simulink model "F16nonlin_K_q"  (R2023b)
settings: Solver=ode4  StartTime=0  StopTime=5  FixedStep=0.01  RelTol=1e-3  EnableMultiTasking=on
values from neighbouring files (symbols this model uses):
  C_nl = C(8,:)    [compare_lin_nonlin.m]    (also in plot_Kq_lin_nonlin.m; runsim_K_pqr.m)
  CA_nl = C_nl*A    [compare_lin_nonlin.m]    (also in plot_Kq_lin_nonlin.m; runsim_K_pqr.m)
  fc = 1/2    (= 0.5)    [compare_lin_nonlin.m]    (also in plot_Kq_lin_nonlin.m)
  invCB_nl = inv(CB_nl)    [compare_lin_nonlin.m]    (also in plot_Kq_lin_nonlin.m; runsim_K_pqr.m)
  Kq = 2    [compare_lin_nonlin.m]    (also in plot_Kq_lin_nonlin.m)
  U_trim = [0.154007747083 -0.694801754663 0.00182544197392 0.000329744079809]    [trimcond.mat]
  X_trim = [501.999976668 0.0505473192089 -2.30406790676e-05 0.000102787556036 0.0505344970072 7.11881239542e-07 -0.000134428882921 -3.64533551716e-06 -1.91663482729e-05 0 0 0 ... (13 elements, 13x1)]    [trimcond.mat]
  xcg = 0.35    [trimcond.mat]
settings Model: Creator=keviczky  LastModifiedBy=suvo
settings DataIOCC: Decimation=50  SaveFormat=Array  SignalLoggingSaveFormat=ModelDataLogs  ReturnWorkspaceOutputs=off  SignalLoggingName=sigsOut
settings OptimizationCC: BooleanDataType=off
settings DebuggingCC: SaveWithParameterizedLinksMsg=none  UnderspecifiedInitializationDetection=Classic  MergeDetectMultiDrivingBlocksExec=none  SignalResolutionControl=TryResolveAllWithWarning  MultiTaskDSMMsg=warning  MultiTaskCondExecSysMsg=none  UnconnectedInputMsg=warning  UnconnectedOutputMsg=warning  UnconnectedLineMsg=warning
settings HardwareCC: ProdBitPerPointer=32  ProdBitPerSizeT=32  ProdBitPerPtrDiffT=32  ProdLargestAtomicFloat=None  ProdIntDivRoundTo=Undefined  ProdEndianess=Unspecified  ProdWordSize=32  ProdHWDeviceType=32-bit Generic  TargetUnknown=on
settings ModelReferenceCC: PropagateSignalLabelsOutOfModel=off
settings GRTTargetCC: CombineOutputUpdateFcns=off  GRTInterface=on
settings ConfigComp: CovMetricSettings=dw  CovSaveCumulativeToWorkspaceVar=on  CovSaveSingleToWorkspaceVar=on

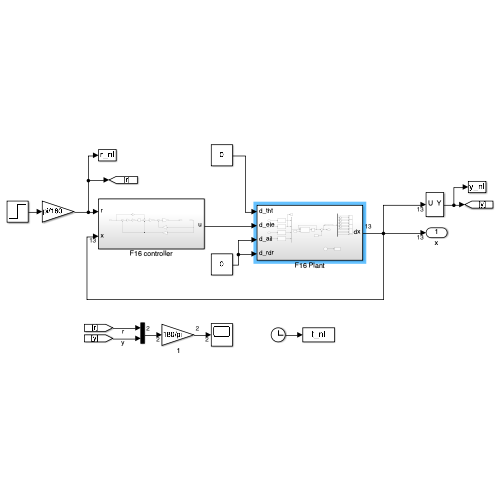
[thumbnail: Simulink's stored preview of the top-level diagram]
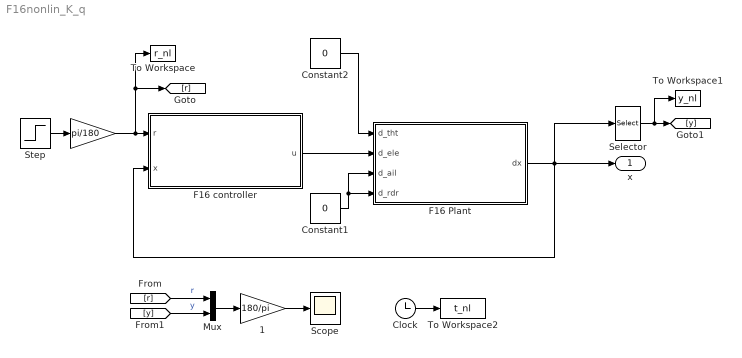
== system F16nonlin_K_q ==
  " " : Gain  Gain=pi/180
  " 1" : Gain  Gain=180/pi
  Clock : Clock
  Constant1 : Constant  Value=0
  Constant2 : Constant  Value=0
  F16 Plant : Subsystem
  F16 controller : Subsystem
  Mux : Mux  Inputs=2
  Scope : Scope
  Selector : Selector  InputPortWidth=13  IndexOptions=Index vector (dialog)  Indices=8  OutputSizes=1
  Step : Step  SampleTime=0
  To Workspace : ToWorkspace  VariableName=r_nl  SampleTime=-1
  To Workspace1 : ToWorkspace  VariableName=y_nl  SampleTime=-1
  To Workspace2 : ToWorkspace  VariableName=t_nl  SampleTime=-1
  x : Outport
  wires:
  Constant2/1 -> F16 Plant/1(d_tht)
  Step/1 -> " "/1
  [r] -> Mux/1  "r"
  [y] -> Mux/2  "y"
  Mux/1 -> " 1"/1
  Selector/1 -> To Workspace1/1, [y]
  " "/1 -> F16 controller/1(r), To Workspace/1, [r]
  " 1"/1 -> Scope/1
  Clock/1 -> To Workspace2/1
  Constant1/1 -> F16 Plant/4(d_rdr), F16 Plant/3(d_ail)
  F16 Plant/1(dx) -> F16 controller/2(x), Selector/1, x/1
  F16 controller/1(u) -> F16 Plant/2(d_ele)

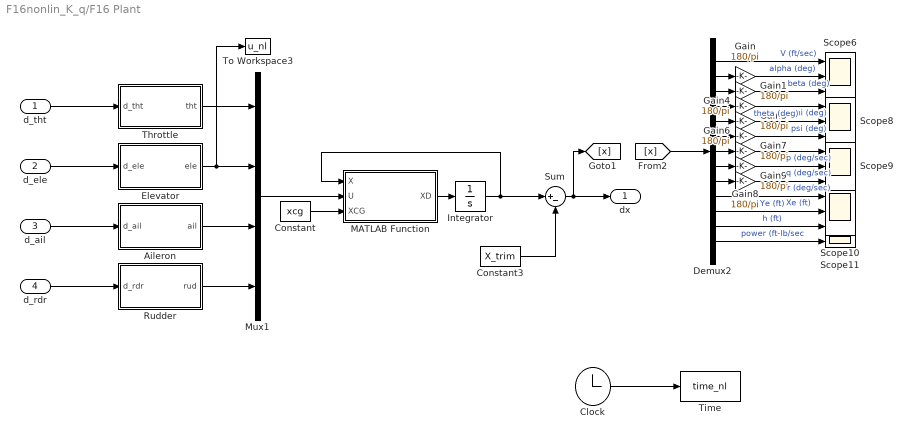
== system F16nonlin_K_q/F16 Plant ==
  d_tht : Inport
  d_ele : Inport  Port=2
  d_ail : Inport  Port=3
  d_rdr : Inport  Port=4
  Aileron : Subsystem
  Clock : Clock
  Constant : Constant  Value=xcg
  Constant3 : Constant  Value=X_trim
  Demux2 : Demux  Outputs=13
  Elevator : Subsystem
  Gain{,1,4..9} (8 alike) : Gain  Gain=180/pi
  Integrator : Integrator  InitialCondition=X_trim
  MATLAB Function : MATLAB Function  TreatAsAtomicUnit=on
  Mux1 : Mux
  Rudder : Subsystem
  Scope{6,8..10} (4 alike) : Scope  NumInputPorts=3
  Scope11 : Scope
  Sum : Sum  Inputs=|+-
  Throttle : Subsystem
  Time : ToWorkspace  VariableName=time_nl  SampleTime=-1
      settings: Decimation=100
  To Workspace3 : ToWorkspace  VariableName=u_nl  SampleTime=-1
  dx : Outport
  wires:
  Demux2/7 -> Gain7/1
  Demux2/11 -> Scope10/2  "Ye (ft)"
  Demux2/2 -> Gain/1
  Demux2/10 -> Scope10/1  "Xe (ft)"
  Integrator/1 -> Sum/1, MATLAB Function/1(X)
  MATLAB Function/1(XD) -> Integrator/1
  Gain4/1 -> Scope8/1  "phi (deg)"
  Demux2/5 -> Gain5/1
  Gain6/1 -> Scope8/3  "psi (deg)"
  Gain/1 -> Scope6/2  "alpha (deg)"
  Demux2/8 -> Gain8/1
  Gain8/1 -> Scope9/2  "q (deg/sec)"
  Mux1/1 -> MATLAB Function/2(U)
  Gain9/1 -> Scope9/3  "r (deg/sec)"
  Demux2/6 -> Gain6/1
  Demux2/3 -> Gain1/1
  Demux2/12 -> Scope10/3  "h (ft)"
  Clock/1 -> Time/1
  Gain1/1 -> Scope6/3  "beta (deg)"
  Demux2/13 -> Scope11/1  "power (ft-lb/sec"
  Demux2/1 -> Scope6/1  "V (ft/sec)"
  Gain7/1 -> Scope9/1  "p (deg/sec)"
  Constant/1 -> MATLAB Function/3(XCG)
  [x] -> Demux2/1
  Demux2/9 -> Gain9/1
  Demux2/4 -> Gain4/1
  Gain5/1 -> Scope8/2  "theta (deg)"
  Throttle/1(tht) -> Mux1/1
  Elevator/1(ele) -> To Workspace3/1, Mux1/2
  Aileron/1(ail) -> Mux1/3
  Rudder/1(rud) -> Mux1/4
  d_rdr/1 -> Rudder/1(d_rdr)
  d_ail/1 -> Aileron/1(d_ail)
  d_ele/1 -> Elevator/1(d_ele)
  d_tht/1 -> Throttle/1(d_tht)
  Sum/1 -> [x], dx/1
  Constant3/1 -> Sum/2

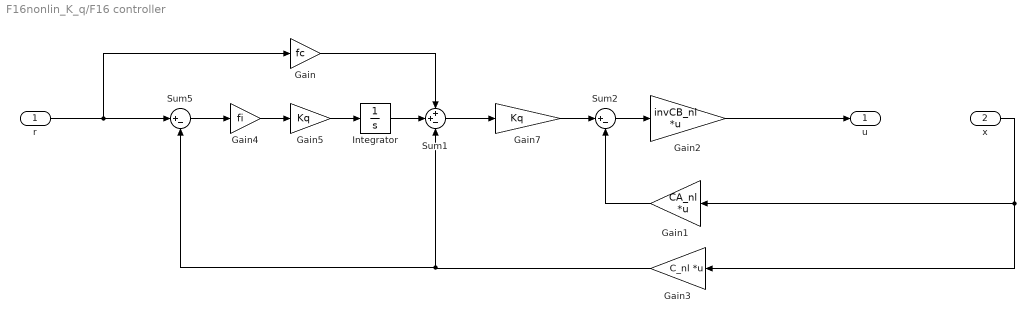
== system F16nonlin_K_q/F16 controller ==
  r : Inport
  x : Inport  Port=2
  Gain : Gain  Gain=fc
  Gain1 : Gain  Gain=CA_nl  Multiplication=Matrix(K*u)
  Gain2 : Gain  Gain=invCB_nl  Multiplication=Matrix(K*u)
  Gain3 : Gain  Gain=C_nl  Multiplication=Matrix(K*u)
  Gain4 : Gain  Gain=fi
  Gain5 : Gain  Gain=Kq
  Gain7 : Gain  Gain=Kq
  Integrator : Integrator
  Sum1 : Sum  Inputs=++-
  Sum2 : Sum  Inputs=|+-
  Sum5 : Sum  Inputs=|+-
  u : Outport
  wires:
  Gain2/1 -> u/1
  Sum1/1 -> Gain7/1
  r/1 -> Gain/1, Sum5/1
  x/1 -> Gain3/1, Gain1/1
  Gain5/1 -> Integrator/1
  Sum2/1 -> Gain2/1
  Gain1/1 -> Sum2/2
  Gain/1 -> Sum1/1
  Sum5/1 -> Gain4/1
  Gain4/1 -> Gain5/1
  Gain3/1 -> Sum1/3, Sum5/2
  Gain7/1 -> Sum2/1
  Integrator/1 -> Sum1/2

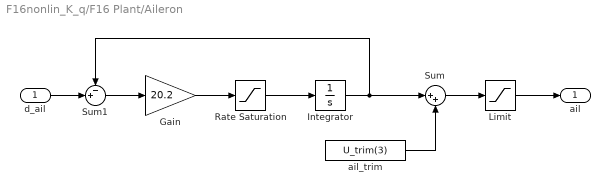
== system F16nonlin_K_q/F16 Plant/Aileron ==
  d_ail : Inport
  Gain : Gain  Gain=20.2  SaturateOnIntegerOverflow=on  OutDataTypeStr=Inherit: Same as input  ParamDataTypeStr=Inherit: Same as input
  Integrator : Integrator  UpperSaturationLimit=25  LowerSaturationLimit=-25
  Limit : Saturate  UpperLimit=25  LowerLimit=-25
  Rate Saturation : Saturate  UpperLimit=60  LowerLimit=-60
  Sum : Sum  Inputs=|++  InputSameDT=on  SaturateOnIntegerOverflow=on  OutDataTypeStr=Inherit: Same as first input
  Sum1 : Sum  Inputs=-+|  InputSameDT=on  SaturateOnIntegerOverflow=on  OutDataTypeStr=Inherit: Same as first input
  ail_trim : Constant  Value=U_trim(3)
  ail : Outport
  wires:
  Sum1/1 -> Gain/1
  Gain/1 -> Rate Saturation/1
  Rate Saturation/1 -> Integrator/1
  Integrator/1 -> Sum/1, Sum1/1
  Sum/1 -> Limit/1
  Limit/1 -> ail/1
  ail_trim/1 -> Sum/2
  d_ail/1 -> Sum1/2

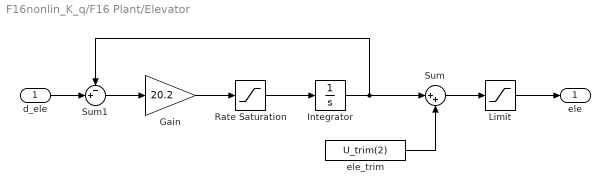
== system F16nonlin_K_q/F16 Plant/Elevator ==
  d_ele : Inport
  Gain : Gain  Gain=20.2  SaturateOnIntegerOverflow=on  OutDataTypeStr=Inherit: Same as input  ParamDataTypeStr=Inherit: Same as input
  Integrator : Integrator  UpperSaturationLimit=25  LowerSaturationLimit=-25
  Limit : Saturate  UpperLimit=25  LowerLimit=-25
  Rate Saturation : Saturate  UpperLimit=60  LowerLimit=-60
  Sum : Sum  Inputs=|++  InputSameDT=on  SaturateOnIntegerOverflow=on  OutDataTypeStr=Inherit: Same as first input
  Sum1 : Sum  Inputs=-+|  InputSameDT=on  SaturateOnIntegerOverflow=on  OutDataTypeStr=Inherit: Same as first input
  ele_trim : Constant  Value=U_trim(2)
  ele : Outport
  wires:
  Sum1/1 -> Gain/1
  Gain/1 -> Rate Saturation/1
  Rate Saturation/1 -> Integrator/1
  Integrator/1 -> Sum/1, Sum1/1
  Sum/1 -> Limit/1
  Limit/1 -> ele/1
  ele_trim/1 -> Sum/2
  d_ele/1 -> Sum1/2

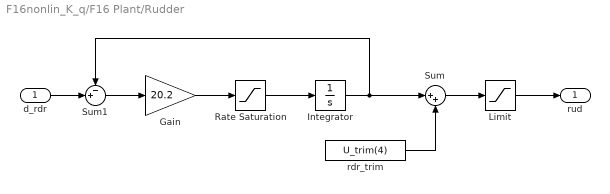
== system F16nonlin_K_q/F16 Plant/Rudder ==
  d_rdr : Inport
  Gain : Gain  Gain=20.2  SaturateOnIntegerOverflow=on  OutDataTypeStr=Inherit: Same as input  ParamDataTypeStr=Inherit: Same as input
  Integrator : Integrator  UpperSaturationLimit=25  LowerSaturationLimit=-25
  Limit : Saturate  UpperLimit=25  LowerLimit=-25
  Rate Saturation : Saturate  UpperLimit=60  LowerLimit=-60
  Sum : Sum  Inputs=|++  InputSameDT=on  SaturateOnIntegerOverflow=on  OutDataTypeStr=Inherit: Same as first input
  Sum1 : Sum  Inputs=-+|  InputSameDT=on  SaturateOnIntegerOverflow=on  OutDataTypeStr=Inherit: Same as first input
  rdr_trim : Constant  Value=U_trim(4)
  rud : Outport
  wires:
  Sum1/1 -> Gain/1
  Gain/1 -> Rate Saturation/1
  Rate Saturation/1 -> Integrator/1
  Integrator/1 -> Sum/1, Sum1/1
  Sum/1 -> Limit/1
  Limit/1 -> rud/1
  rdr_trim/1 -> Sum/2
  d_rdr/1 -> Sum1/2

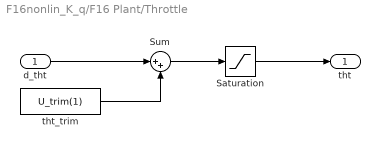
== system F16nonlin_K_q/F16 Plant/Throttle ==
  d_tht : Inport
  Saturation : Saturate  UpperLimit=1  LowerLimit=0
  Sum : Sum  Inputs=|++  InputSameDT=on  SaturateOnIntegerOverflow=on  OutDataTypeStr=Inherit: Same as first input
  tht_trim : Constant  Value=U_trim(1)
  tht : Outport
  wires:
  Sum/1 -> Saturation/1
  Saturation/1 -> tht/1
  d_tht/1 -> Sum/1
  tht_trim/1 -> Sum/2

== matlab function F16nonlin_K_q/F16 Plant/MATLAB Function ==
  data: X input; U input; XD output; XCG input
function XD = F16DYN(X,U,XCG)
% f16 dynamics

% Author: Subhabrata Ganguli
%
% Ref: Stevens, Brian L.; Lewis, Frank L.; Johnson, Eric N.. 
% Aircraft Control and Simulation: Dynamics, 
% Controls Design, and Autonomous Systems. 
% Wiley.

%% Parameters

AXX = 9496.0;
AYY = 55814.0;
AZZ = 63100.0;
AXZ =   982.0;

AXZS = AXZ^2;
XPQ  = AXZ * (AXX - AYY + AZZ);
GAM = AXX * AZZ - AXZ^2;

XQR = AZZ * (AZZ - AYY) + AXZS;
ZPQ =(AXX-AYY) * AXX + AXZS;
YPR = AZZ - AXX;

WEIGHT = 25000.0;
GD = 32.174;
MASS = WEIGHT/GD;

S = 300;
B = 30;
CBAR = 11.32;
XCGR = 0.35;
HX = 160;
RTOD = 180/pi;

%% Assign State and Control Variables

VT = X(1); 
ALPHA = X(2)*RTOD; 
BETA = X(3)*RTOD;
PHI = X(4); 
THETA = X(5); 
PSI = X(6);
P = X(7); 
Q = X(8); 
R = X(9); 
ALT = X(12); 
POW = X(13);

THTL = U(1);
EL = U(2);
AIL = U(3);
RDR = U(4);

XD = zeros(13,1);

%% Air data computer and engine model

[TFAC, T, RHO, AMACH, QBAR, PS ] = ADC (VT, ALT);
CPOW = TGEAR(THTL);

XD(13) = PDOT(POW,CPOW);     
T = THRUST(POW,ALT,AMACH);

%% Look-up tables and component buildup

CXT = CX (ALPHA,EL);
CYT = CY (BETA,AIL,RDR);
CZT = CZ (ALPHA,BETA,EL);
      
DAIL= AIL/20.0; DRDR= RDR/30.0;

DLDA_OUT = DLDA(ALPHA,BETA);
DLDR_OUT = DLDR(ALPHA,BETA);
DNDA_OUT = DNDA(ALPHA,BETA);
DNDR_OUT = DNDR(ALPHA,BETA);

CLT = CL(ALPHA,BETA) + DLDA_OUT*DAIL + DLDR_OUT*DRDR;
CMT = CM(ALPHA,EL);
CNT = CN(ALPHA,BETA) + DNDA_OUT*DAIL + DNDR_OUT*DRDR;

%% Add damping derivatives

TVT = 0.5/VT; 
B2V = B*TVT; 
CQ = CBAR*Q*TVT;

D = DAMP(ALPHA);

CXT = CXT + CQ * D(1);
CYT = CYT + B2V * ( D(2)*R + D(3)*P );
CZT = CZT + CQ * D(4);
CLT = CLT + B2V * ( D(5)*R + D(6)*P );
CMT = CMT + CQ * D(7) + CZT * (XCGR-XCG);
CNT = CNT + B2V*(D(8)*R + D(9)*P) - CYT*(XCGR-XCG) * CBAR/B;

%% Get ready for state equations

CBTA  = cos(X(3)); 
U     = VT*cos(X(2))*CBTA;
V     = VT * sin(X(3)); 
W     = VT*sin(X(2))*CBTA;
STH   = sin(THETA); 
CTH   = cos(THETA);   
SPH   = sin(PHI);
CPH   = cos(PHI); 
SPSI  = sin(PSI);    
CPSI  = cos(PSI);
QS    = QBAR * S; 
QSB   = QS * B;        
RMQS  = QS/MASS;
GCTH  = GD * CTH; 
QSPH  = Q * SPH;
AY    = RMQS*CYT; 
AZ    = RMQS * CZT;

%% Force Equations

UDOT   = R*V - Q*W - GD*STH + (QS * CXT + T)/MASS;
VDOT   = P*W - R*U + GCTH * SPH + AY;
WDOT   = Q*U - P*V + GCTH * CPH + AZ;
    
DUM   = (U*U + W*W);
XD(1) = (U*UDOT + V*VDOT + W*WDOT)/VT;
XD(2) = (U*WDOT - W*UDOT) / DUM;
XD(3) = (VT*VDOT- V*XD(1)) * CBTA / DUM;

%% Kinematics

XD(4) = P + (STH/CTH)*(QSPH + R*CPH);
XD(5) = Q*CPH - R*SPH;
XD(6) = (QSPH + R*CPH)/CTH;

%% Moments

ROLL  = QSB*CLT;
PITCH = QS *CBAR*CMT;
YAW   = QSB*CNT;
PQ    = P*Q;
QR    = P*R;
QHX   = Q*HX;
XD(7) = ( XPQ*PQ - XQR*QR + AZZ*ROLL + AXZ*(YAW + QHX) )/GAM;
XD(8) = ( YPR*P*R - AXZ*(P^2 - R^2) + PITCH - R*HX )/AYY;
XD(9) = ( ZPQ*PQ - XPQ*QR + AXZ*ROLL + AXX*(YAW + QHX) )/GAM;

%% Navigation

T1 = SPH * CPSI; 
T2 = CPH * STH; 
T3 = SPH * SPSI;
S1 = CTH * CPSI; 
S2 = CTH * SPSI; 
S3 = T1 * STH - CPH * SPSI;
S4 = T3 * STH + CPH * CPSI; 
S5 = SPH * CTH; 
S6 = T2 * CPSI + T3;
S7 = T2 * SPSI - T1; 
S8 = CPH * CTH;

XD(10)  = U * S1 + V * S3 + W * S6;   %   North speed
XD(11)  = U * S2 + V * S4 + W * S7;   %   East speed
XD(12)  = U * STH -V * S5 - W * S8;   %   Vertical speed

XD = XD(:);

end
